simulink model "buck_boost_l2"  (R2023a)
settings: Solver=FixedStepAuto  StartTime=0.0  StopTime=0.5  FixedStep=ts  RelTol=1e-3
values from neighbouring files (symbols this model uses):
  C = 60e-6    (= 6e-05)    [init.m]
  fsw = 25e3    (= 25000)    [init.m]
  ki = 20    [init.m]
  kp = 0    [init.m]
  L = 100e-6    (= 0.0001)    [init.m]
  R = 5    [init.m]
  RC = 2e-3    (= 0.002)    [init.m]
  RL = 10e-3    (= 0.01)    [init.m]
  ts = 1e-6    (= 1e-06)    [init.m]
  vin = 100    [init.m]
libraries: simulink x2
settings Model: Creator=ptrujillo  LastModifiedBy=pablo
settings SolverCC: AlgebraicLoopSolver=TrustRegion
settings DataIOCC: ReturnWorkspaceOutputs=off
settings DebuggingCC: UnconnectedInputMsg=warning  UnconnectedOutputMsg=warning  UnconnectedLineMsg=warning  ArithmeticOperatorsInVariantConditions=warning
settings ModelReferenceCC: EnableRefExpFcnMdlSchedulingChecks=on
settings SFSimCC: CustomCodeUndefinedFunction=UseInterfaceOnly

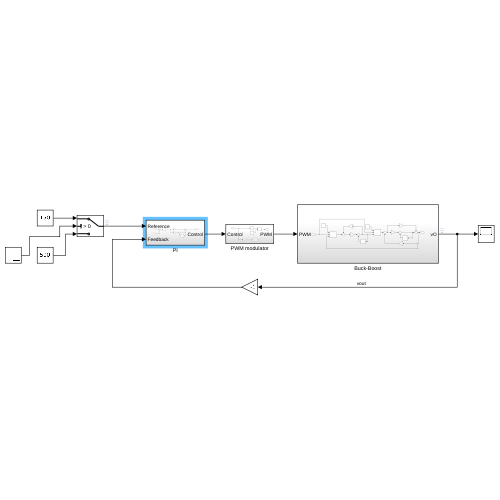
[thumbnail: Simulink's stored preview of the top-level diagram]
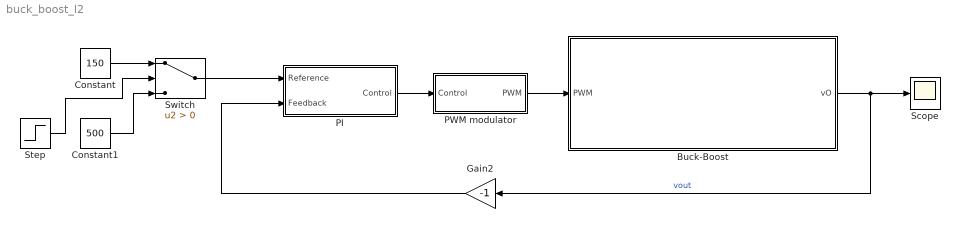
== system buck_boost_l2 ==
  Buck-Boost : Subsystem
  Constant : Constant  Value=150
  Constant1 : Constant  Value=500
  Gain2 : Gain  Gain=-1
  PI : Subsystem
  PWM modulator : Subsystem
  Scope : Scope
  Step : Step  Time=0.2  Before=1  After=0  SampleTime=0
  Switch : Switch  Criteria=u2 > Threshold  SaturateOnIntegerOverflow=off  InputSameDT=off
  wires:
  Buck-Boost/1(vO) -> Gain2/1, Scope/1  "vout"
  Gain2/1 -> PI/2(Feedback)
  PI/1(Control) -> PWM modulator/1(Control)
  PWM modulator/1(PWM) -> Buck-Boost/1("PWM ")
  Constant/1 -> Switch/1
  Switch/1 -> PI/1(Reference)
  Constant1/1 -> Switch/3
  Step/1 -> Switch/2

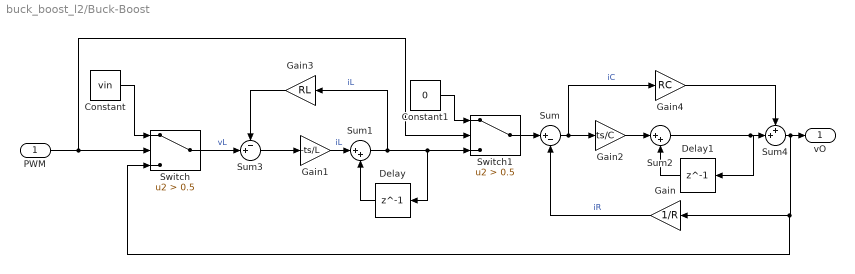
== system buck_boost_l2/Buck-Boost ==
  "PWM " : Inport
  Constant : Constant  Value=vin
  Constant1 : Constant  Value=0
  Delay : Delay  DelayLength=1  SampleTime=ts
  Delay1 : Delay  DelayLength=1  SampleTime=ts
  Gain : Gain  Gain=1/R
  Gain1 : Gain  Gain=-ts/L
  Gain2 : Gain  Gain=ts/C
  Gain3 : Gain  Gain=RL
  Gain4 : Gain  Gain=RC
  Sum : Sum  Inputs=|+-
  Sum1 : Sum  Inputs=|++
  Sum2 : Sum  Inputs=|++
  Sum3 : Sum  Inputs=-+|
  Sum4 : Sum  Inputs=++|
  Switch : Switch  Criteria=u2 > Threshold  Threshold=0.5  SaturateOnIntegerOverflow=off  InputSameDT=off
  Switch1 : Switch  Criteria=u2 > Threshold  Threshold=0.5  SaturateOnIntegerOverflow=off  InputSameDT=off
  vO : Outport  VectorParamsAs1DForOutWhenUnconnected=off
  wires:
  Constant1/1 -> Switch1/1
  Sum1/1 -> Gain3/1, Delay/1, Switch1/3  "iL"
  "PWM "/1 -> Switch1/2, Switch/2
  Sum/1 -> Gain4/1, Gain2/1  "iC"
  Constant/1 -> Switch/1
  Switch1/1 -> Sum/1
  Sum2/1 -> Delay1/1, Sum4/2
  Gain/1 -> Sum/2  "iR"
  Switch/1 -> Sum3/2  "vL"
  Gain1/1 -> Sum1/1  "iL"
  Delay/1 -> Sum1/2
  Gain2/1 -> Sum2/1
  Delay1/1 -> Sum2/2
  Sum3/1 -> Gain1/1
  Gain3/1 -> Sum3/1
  Sum4/1 -> Switch/3, Gain/1, vO/1
  Gain4/1 -> Sum4/1

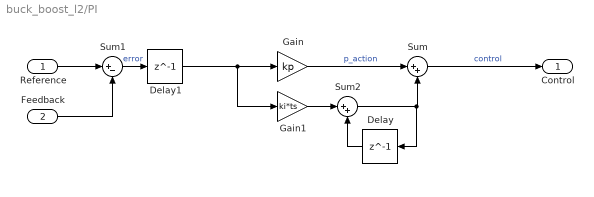
== system buck_boost_l2/PI ==
  Reference : Inport
  Feedback : Inport  Port=2
  Delay : Delay  DelayLength=1
  Delay1 : Delay  DelayLength=1  SampleTime=ts
  Gain : Gain  Gain=kp
  Gain1 : Gain  Gain=ki*ts
  Sum : Sum  Inputs=|++
  Sum1 : Sum  Inputs=|+-
  Sum2 : Sum  Inputs=|++
  Control : Outport  VectorParamsAs1DForOutWhenUnconnected=off
  wires:
  Gain1/1 -> Sum2/1
  Delay/1 -> Sum2/2
  Sum2/1 -> Delay/1, Sum/2
  Sum/1 -> Control/1  "control"
  Feedback/1 -> Sum1/2
  Sum1/1 -> Delay1/1  "error"
  Reference/1 -> Sum1/1
  Delay1/1 -> Gain1/1, Gain/1
  Gain/1 -> Sum/1  "p_action"

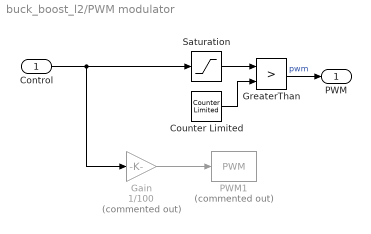
== system buck_boost_l2/PWM modulator ==
  Control : Inport
  Counter Limited : simulink/Sources/Counter Limited  uplimit=100  tsamp=-1
  Gain : Gain  Commented=on  Gain=1/100
  GreaterThan : RelationalOperator  Operator=>  OutDataTypeStr=boolean  RndMeth=Simplest  InputSameDT=off
  PWM1 : simulink/Discontinuities/PWM  Commented=on  DisableCoverage=on  Period=1/fsw  InitialDelay=0  DisallowZeroDutyCycle=off  RunAtFixedTimeIntervals=on  SampleTime=ts
  Saturation : Saturate  UpperLimit=90  LowerLimit=0
  PWM : Outport  VectorParamsAs1DForOutWhenUnconnected=off
  wires:
  Saturation/1 -> GreaterThan/1
  Counter Limited/1 -> GreaterThan/2
  Control/1 -> Saturation/1, Gain/1
  Gain/1 -> PWM1/1
  GreaterThan/1 -> PWM/1  "pwm"
